simulink model "pump_4"  (R2018b)
settings: Solver=ode45  StartTime=0.0  StopTime=600  MaxStep=10  RelTol=1e-3  EnableMultiTasking=on
undefined symbols (not defined in the file): path_carnot
libraries: carnot x8, simulink x1
settings Model: Creator=drhf  LastModifiedBy=drhf
settings SolverCC: ZeroCrossAlgorithm=Adaptive
settings DataIOCC: LimitDataPoints=on  SaveFormat=Array  SignalLoggingSaveFormat=ModelDataLogs
settings OptimizationCC: ExpressionDepthLimit=2147483647  LifeSpan=inf
settings DebuggingCC: UnderspecifiedInitializationDetection=Classic  MergeDetectMultiDrivingBlocksExec=none  IgnoredZcDiagnostic=none  SolverPrmCheckMsg=warning  FcnCallInpInsideContextMsg=warning  StateNameClashWarn=warning  SFUnexpectedBacktrackingDiag=warning  SFNoUnconditionalDefaultTransitionDiag=warning  SFExecutionAtInitializationDiag=none
settings HardwareCC: ProdBitPerPointer=32  ProdBitPerSizeT=32  ProdBitPerPtrDiffT=32  ProdLargestAtomicFloat=None  ProdIntDivRoundTo=Undefined  ProdEndianess=Unspecified  ProdWordSize=32  ProdHWDeviceType=32-bit Generic
settings ModelReferenceCC: PropagateSignalLabelsOutOfModel=off
settings SFSimCC: SimUseLocalCustomCode=off
settings RTWCC: RTWUseLocalCustomCode=off
settings CodeAppCC: StateflowObjectComments=on
settings GRTTargetCC: TargetLangStandard=C89/C90 (ANSI)  GeneratePreprocessorConditionals=Disable all  CombineOutputUpdateFcns=off  GRTInterface=on
settings ConfigComp: CovMetricSettings=dw  CovHtmlReporting=on  CovSaveCumulativeToWorkspaceVar=on  CovSaveSingleToWorkspaceVar=on  CovExternalEMLEnable=off

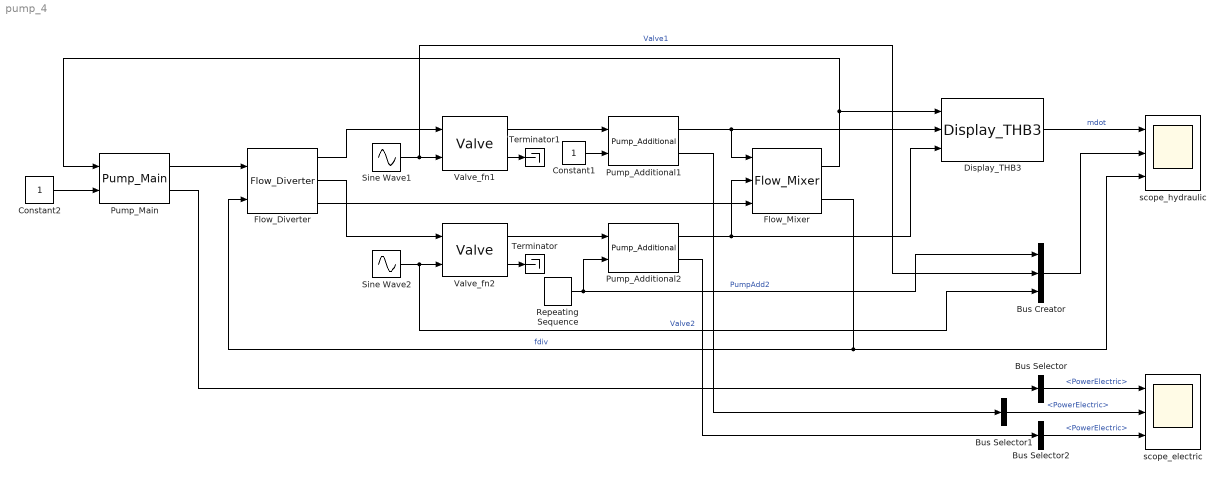
== system pump_4 ==
  Bus Creator : BusCreator  Inputs=3
  Bus Selector : BusSelector  OutputSignals=PowerElectric
  Bus Selector1 : BusSelector  OutputSignals=PowerElectric
  Bus Selector2 : BusSelector  OutputSignals=PowerElectric
  Constant1 : Constant
  Constant2 : Constant
  Display_THB3 : carnot/Outputs/Display_THB3  t=off  m=on  p=off  id=off  mix=off  d=off
  Flow_Diverter : carnot/Hydraulics/Flow_Diverter
  Flow_Mixer : carnot/Hydraulics/Flow_Mixer
  Pump_Additional1 : carnot/Hydraulics/Pump_Additional  Tini=20  PathName=fullfile(path_carnot('libsl'), 'Hydraulics', 'Pump_Main', 'parameter_set')  FileName='Pump6m.mat'  userPath=off  userParam=off  a0=60000  a1=-43200  a2=0  dia=0.025  UA=1  mcp=4182  e0=50  e1=28.8  e2=-10.368
  Pump_Additional2 : carnot/Hydraulics/Pump_Additional  Tini=20  PathName=fullfile(path_carnot('libsl'), 'Hydraulics', 'Pump_Main', 'parameter_set')  FileName='Pump6m.mat'  userPath=off  userParam=off  a0=60000  a1=-43200  a2=0  dia=0.025  UA=1  mcp=4182  e0=50  e1=28.8  e2=-10.368
  Pump_Main : carnot/Hydraulics/Pump_Main  Tini=20  p0=2e5  IDpreset=pressure drop  fluid=Water  mix=0  mix2=0  mix3=0  t1=0.1  PathName=fullfile(path_carnot('libsl'), 'Hydraulics', 'Pump_Main', 'parameter_set')  FileName='Pump6m.mat'  userPath=off  userParam=off  a0=60000  a1=-43200  a2=0  dia=0.025  UA=1  mcp=4182  e0=50  e1=28.8  e2=-10.368
  Repeating Sequence : simulink/Sources/Repeating Sequence  rep_seq_t=[0 10 20 278 280 290 300 600]  rep_seq_y="[0  0   1    1     0   0    1     1]"
  Sine Wave1 : Sin  Amplitude=0.6  Bias=0.5  Frequency=1/60  SampleTime=0
  Sine Wave2 : Sin  Amplitude=0.6  Bias=0.5  Frequency=1/60  Phase=pi  SampleTime=0
  Terminator : Terminator
  Terminator1 : Terminator
  Valve_fn1 : carnot/Hydraulics/Valve  vtyp=linear  psi_0=0.04  kvs=0.9  dt_V=30
  Valve_fn2 : carnot/Hydraulics/Valve  vtyp=linear  psi_0=0.04  kvs=0.9  dt_V=30
  scope_electric : Scope  NumInputPorts=3
  scope_hydraulic : Scope  NumInputPorts=3
  wires:
  Constant2/1 -> Pump_Main/2
  Sine Wave1/1 -> Valve_fn1/2, Bus Creator/2  "Valve1"
  Pump_Main/1 -> Flow_Diverter/1
  Flow_Diverter/1 -> Valve_fn1/1
  Sine Wave2/1 -> Valve_fn2/2, Bus Creator/3  "Valve2"
  Flow_Diverter/2 -> Valve_fn2/1
  Flow_Diverter/3 -> Flow_Mixer/3
  Flow_Mixer/2 -> scope_hydraulic/3, Flow_Diverter/2  "fdiv"
  Flow_Mixer/1 -> Pump_Main/1, Display_THB3/1
  Display_THB3/1 -> scope_hydraulic/1  "mdot"
  Bus Creator/1 -> scope_hydraulic/2
  Valve_fn2/1 -> Pump_Additional2/1
  Pump_Additional2/1 -> Flow_Mixer/2, Display_THB3/3
  Pump_Additional2/2 -> Bus Selector2/1
  Repeating Sequence/1 -> Bus Creator/1, Pump_Additional2/2  "PumpAdd2"
  Valve_fn1/1 -> Pump_Additional1/1
  Constant1/1 -> Pump_Additional1/2
  Pump_Additional1/1 -> Display_THB3/2, Flow_Mixer/1
  Pump_Additional1/2 -> Bus Selector1/1
  Pump_Main/2 -> Bus Selector/1
  Bus Selector/1 -> scope_electric/1  "<PowerElectric>"
  Bus Selector1/1 -> scope_electric/2  "<PowerElectric>"
  Bus Selector2/1 -> scope_electric/3  "<PowerElectric>"
  Valve_fn2/2 -> Terminator/1
  Valve_fn1/2 -> Terminator1/1
